simulink model "HW02_96101838_4_2"  (R2017a)
settings: Solver=VariableStepAuto  StartTime=0.0  StopTime=600  RelTol=1e-3
settings Model: Creator=Micronet  LastModifiedBy=Micronet

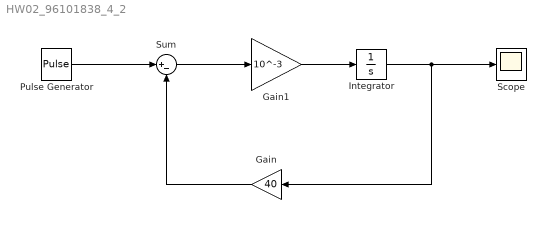
== system HW02_96101838_4_2 ==
  Gain : Gain  Gain=40
  Gain1 : Gain  Gain=10^-3
  Integrator : Integrator
  Pulse Generator : DiscretePulseGenerator  PulseType=Time based  Amplitude=400  Period=300  PulseWidth=20
  Scope : Scope
  Sum : Sum  Inputs=|+-
  wires:
  Sum/1 -> Gain1/1
  Gain1/1 -> Integrator/1
  Integrator/1 -> Gain/1, Scope/1
  Gain/1 -> Sum/2
  Pulse Generator/1 -> Sum/1
